simulink model "Robot_Sim"  (R2018a)
settings: Solver=ode45  StartTime=0.0  StopTime=Tsim  FixedStep=Ts_compute  RelTol=1e-3
values from neighbouring files (symbols this model uses):
  A_enc = [1 -Ts_sensor;0 1]    [Model.m]
  A_g = [1 -Ts_sensor;0 1]    [Model.m]
  A_y = [1 Ts_sensor Ts_sensor^2/2 ... (first row only)    [Model.m]
  B_enc = [Ts_sensor 0]'    [Model.m]
  B_g = [Ts_sensor 0]'    [Model.m]
  buffer_size = 15    [Model.m]
  C_enc = [1 0]    [Model.m]
  C_g = [1 0]    [Model.m]
  C_y = [0 0 1]    [Model.m]
  D_den = [1 2*D_WN*D_QSI D_WN^2]    [Model.m]
  D_num = D_WN^2    (= 81)    [Model.m]
  D_rodas = 0.4    [Model.m]
  Di_angle = pi/6    (= 0.523598775598)    [Model.m]
  Di_den = [1 2*Di_WN*Di_QSI Di_WN^2]    [Model.m]
  Di_num = Di_WN^2    (= 9)    [Model.m]
  Di_time = (2.5)*Tsim/8    (= 25)    [Model.m]
  discriminator = 0.8    [Model.m]
  g = u(7)    [ControllerK.m]    (also in Klankar_Marcus.m = 40; LQR.m = 40; Model.m = 40)
  Gyro_bias = 0.004    [Model.m]
  Kd = 0    [Model.m]
  Ki = 10.0    (= 10)    [Model.m]
  Kp = 5.0    (= 5)    [Model.m]
  ksi = u(6)    [ControllerK.m]    (also in Klankar_Marcus.m = 0.3; LQR.m = 0.3; Model.m = 0.6)
  Rv_enc = 0.002    [Model.m]
  Rv_g = 0.020    (= 0.02)    [Model.m]
  Rv_y = 0.01    [Model.m]
  Rw_enc = 0.1*[Ts_sensor^2/2 0;0 Ts_sensor^2/2]    [Model.m]
  Rw_g = 0.01*[Ts_sensor^2/2 0;0 Ts_sensor]    [Model.m]
  Rw_y = 0.05*[Ts_sensor^5/20 Ts_sensor^4/8 Ts_sensor^3/6 ... (first row only)    [Model.m]
  SELETOR_CONTROLADOR = 3    [Model.m]
  Time = 0:Ts:(time-1)*Ts    [InterfaceBT.m]
  Ts = 0.1    [InterfaceBT.m]    (also in Klankar_Marcus.m; LQR.m; Model.m)
  Ts_sensor = 1/50    (= 0.02)    [Model.m]
  Tsim = 70    [Klankar_Marcus.m]    (also in LQR.m = 63; Model.m = 80)
  V_MAX = 1    [Model.m]
  V_WHEEL_MAX = 1    [Model.m]
  W_MAX = 1    [Model.m]
undefined symbols (not defined in the file or in its folder): Controlador_LPV, DiscIntNeverNeededParam, Discrete, K_KALM_g, K_LQ
libraries: simulink x8, ctrlSharedLib x2, cstblocks x2
settings Model: PauseTimes=28  NumberOfSteps=10  Creator=davi2  LastModifiedBy=marcus
settings OptimizationCC: LifeSpan=inf
settings DebuggingCC: SFExecutionAtInitializationDiag=none
settings HardwareCC: ProdBitPerSizeT=32  ProdBitPerPtrDiffT=32  ProdWordSize=32  ProdHWDeviceType=Specified
settings CodeAppCC: StateflowObjectComments=on
settings SimscapeCC: SimscapeNormalizeSystem=off

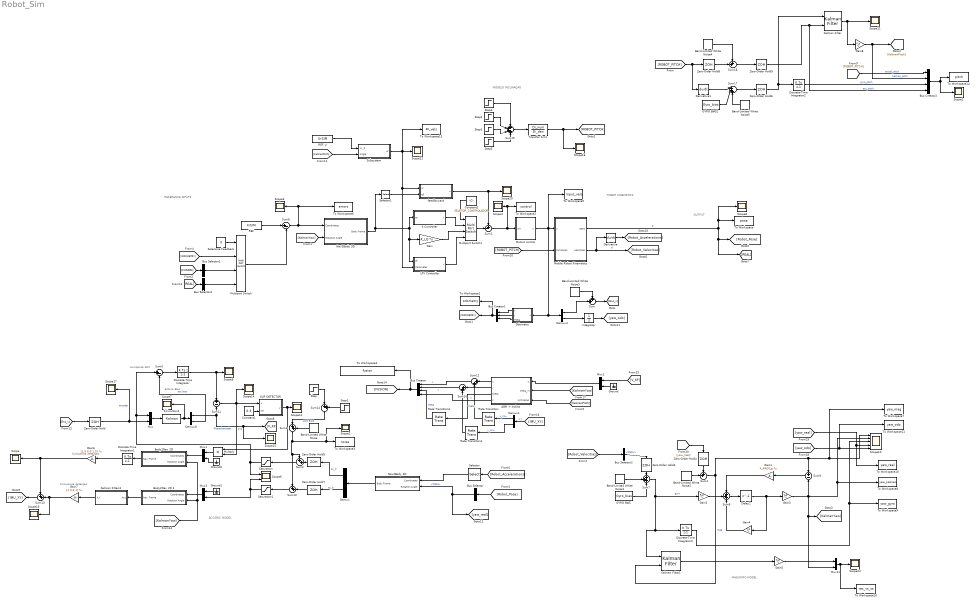
== system Robot_Sim ==
  note: MODELO INCLINAÇAO
  note: Compensa detecçao
  note: estima Bias
  note: compensa ACC
  note: OUTPUT
  note: ROBOT KINEMATICS
  note: MAG/GYRO MODEL
  note: ACC/ENC MODEL
  note: REFERENCE INPUTS
  note: Compensa detecçao
  AGM + Inclina : Subsystem
  Band-Limited White Noise : simulink/Sources/Band-Limited White Noise  Cov=Rv_y^2  Ts=Ts_sensor  seed=[23341]
  Band-Limited White Noise1 : simulink/Sources/Band-Limited White Noise  Cov=Rw_g(1,1)*Rw_g(1,1)  Ts=Ts_sensor  seed=[23341]
  Band-Limited White Noise2 : simulink/Sources/Band-Limited White Noise  Cov=Rv_g^2  Ts=Ts_sensor  seed=[23341]
  Band-Limited White Noise3 : simulink/Sources/Band-Limited White Noise  Cov=Rv_enc^2  Ts=Ts_sensor  seed=[23341]
  Band-Limited White Noise4 : simulink/Sources/Band-Limited White Noise  Cov=Rv_g^2  Ts=Ts_sensor  seed=[23341]
  Band-Limited White Noise5 : simulink/Sources/Band-Limited White Noise  Cov=Rw_g(1,1)*Rw_g(1,1)  Ts=Ts_sensor  seed=[23341]
  Body2Nav 2D : Subsystem
  Body2Nav 2D 2 : Subsystem
  Bus Creator : BusCreator  Inputs=4
  Bus Creator1 : BusCreator  Inputs=3
  Bus Creator2 : BusCreator  Inputs=4
  Bus Selector : BusSelector  OutputSignals=theta
  Bus Selector1 : BusSelector  OutputSignals=x,y,theta  OutputAsBus=on
  Bus Selector2 : BusSelector  OutputSignals=theta'
  Bus Selector3 : BusSelector  OutputSignals=x,y,theta  OutputAsBus=on
  Constant1 : Constant  Value=0.3
  Constant2 : Constant  Value=SELETOR_CONTROLADOR
  Delay2 : Delay  DelayLength=1
  Demux{,1,4,8} (4 alike) : Demux  Outputs=2
  Derivative : Derivative  CoefficientInTFapproximation=1
  Derivative1 : Derivative
  Discrete-Time Integrator : DiscreteIntegrator  IntegratorMethod=Integration: Backward Euler  SampleTime=Ts_sensor  ICPrevOutput=DiscIntNeverNeededParam  ICPrevScaledInput=DiscIntNeverNeededParam
  Discrete-Time Integrator1 : DiscreteIntegrator  SampleTime=Ts_sensor  ICPrevOutput=DiscIntNeverNeededParam  ICPrevScaledInput=DiscIntNeverNeededParam
  Discrete-Time Integrator2 : DiscreteIntegrator  SampleTime=-1  ICPrevOutput=DiscIntNeverNeededParam  ICPrevScaledInput=DiscIntNeverNeededParam
  Discrete-Time Integrator3 : DiscreteIntegrator  SampleTime=-1  ICPrevOutput=DiscIntNeverNeededParam  ICPrevScaledInput=DiscIntNeverNeededParam
  GYRO BIAS : Constant  Value=Gyro_bias
  GYRO BIAS1 : Constant  Value=Gyro_bias
  Gain : Gain  Gain=-K_LQ  Multiplication=Matrix(K*u)
  Gain1 : Gain  Gain=K_KALM_g  Multiplication=Matrix(K*u)
  Gain2 : Gain  Gain=B_g  Multiplication=Matrix(K*u)
  Gain3 : Gain  Gain=C_g  Multiplication=Matrix(K*u)
  Gain4 : Gain  Gain=A_g  Multiplication=Matrix(K*u)
  Gain5 : Gain  Gain=C_g  Multiplication=Matrix(K*u)
  Gain6 : Gain  Gain=[1.5 0;0 1.5]  Multiplication=Matrix(K*u)
  Gain7 : Gain  Gain=[1 0;0 1]  Multiplication=Matrix(K*u)
  Gain8 : Gain  Gain=C_g  Multiplication=Matrix(K*u)
  Ground : Ground
  Ground1 : Ground
  Ground2 : Ground
  Integrator : Integrator
  K Controller : Subsystem
  Kalman Filter : ctrlSharedLib/Kalman Filter  TimeDomain=Discrete-Time  UseCurrentEstimator=on  ModelSource=Individual A, B, C, D matrices  ModelSourceVariable=ss(0.95,1,1,0,1)  A=A_g  B=B_g  C=C_g  D=0  NumberOfStates=1  NumberOfInputs=1  NumberOfOutputs=1  InitialEstimateSource=Dialog  X0=0  P0=10  UseK=off  UseGH=off  NumberOfProcessNoiseInputs=1  G=1  TimeInvariantG=on  H=0  TimeInvariantH=on  Q=Rw_g  TimeInvariantQ=on  R=Rv_g  TimeInvariantR=on  N=0  TimeInvariantN=on  AddInputPort=on  AddEnablePort=off  OutputEstimatedY=off  OutputP=off  Ts=Ts_sensor
      settings: SourceProductBaseCode=CT
  Kalman Filter1 : ctrlSharedLib/Kalman Filter  TimeDomain=Discrete-Time  UseCurrentEstimator=on  ModelSource=LTI State-Space Variable  ModelSourceVariable=ss(A_g,B_g,C_g,0,Ts_sensor)  A=0.95  B=1  C=1  D=0  NumberOfStates=1  NumberOfInputs=1  NumberOfOutputs=1  InitialEstimateSource=Dialog  X0=0  P0=10  UseK=off  UseGH=off  NumberOfProcessNoiseInputs=1  G=1  TimeInvariantG=on  H=0  TimeInvariantH=on  Q=Rw_g  TimeInvariantQ=on  R=Rv_g  TimeInvariantR=on  N=0  TimeInvariantN=on  AddInputPort=on  AddEnablePort=off  OutputEstimatedY=off  OutputP=off  Ts=-1
      settings: SourceProductBaseCode=CT
  Kalman Filters1 : Subsystem
  "LPV Controller " : Subsystem
  Mobile Robot Kinematics : Subsystem
  Motors control : Subsystem
  Multiply : Product
  Multiport Switch : MultiPortSwitch
  Multiport Switch1 : MultiPortSwitch
  Mux{,1..3,11} (5 alike) : Mux  Inputs=2
  Nav2Body 2D : Subsystem
  Nav2Body 3D : Subsystem
  Odometry : Subsystem
  REF : FromWorkspace  VariableName=XrSIM  SampleTime=Ts  OutputAfterFinalValue=Holding final value
  REF U : FromWorkspace  VariableName=UrSIM  SampleTime=Ts  OutputAfterFinalValue=Holding final value
  Rate Transition : RateTransition  OutPortSampleTime=Ts
  Rate Transition1 : RateTransition  OutPortSampleTime=Ts
  Rate Transition3 : RateTransition  OutPortSampleTime=Ts
  S-Function2 : S-Function  FunctionName=Kalman  Parameters=Ts_sensor,A_enc,B_enc,C_enc,Rw_enc,Rv_enc  SFunctionDeploymentMode=off  EnableBusSupport=off
  SLIP DETECTOR : MATLAB Function  TreatAsAtomicUnit=on
  Saturation : Saturate  UpperLimit=4*9.8  LowerLimit=-4*9.8
  Saturation1 : Saturate  UpperLimit=4*9.8  LowerLimit=-4*9.8
  Scope{,1..5,7..8,11..12,14..17,19..21,24} (18 alike) : Scope
  Scope10 : Scope  NumInputPorts=5
  Scope6 : Scope  NumInputPorts=2
  Seleciona Feedback : Constant  Value=3
  Selector : Selector  InputPortWidth=3  IndexOptions=Index vector (dialog)  Indices=[1 2]  OutputSizes=1
  Selector1 : Selector  InputPortWidth=3  IndexOptions=Index vector (dialog)  Indices=3  OutputSizes=1
  Step : Step  Time=10  After=0.05  SampleTime=Ts_sensor
  Step1 : Step  Time=30  After=-0.05  SampleTime=Ts_sensor
  Step2 : Step  Time=Di_time+10  After=-Di_angle  SampleTime=0
  Step3 : Step  Time=Di_time+30  After=-Di_angle  SampleTime=0
  Step4 : Step  Time=Di_time  After=Di_angle  SampleTime=0
  Step5 : Step  Time=Di_time+42  After=Di_angle  SampleTime=0
  Subsystem : Subsystem
  Sum{,2,4,10,13,18} (6 alike) : Sum  Inputs=++|
  Sum1 : Sum  Inputs=+-|
  Sum11 : Sum  Inputs=+-
  Sum{3,12,14,16} (4 alike) : Sum  Inputs=|++
  Sum15 : Sum  Inputs=++++
  Sum17 : Sum  Inputs=|+++
  Sum5 : Sum  Inputs=|+-
  Sum6 : Sum  Inputs=|+-
  Sum7 : Sum  Inputs=+++
  Sum8 : Sum  Inputs=+++
  Sum9 : Sum  Inputs=+-
  To Workspace : ToWorkspace  VariableName=pose  SaveFormat=Timeseries  SampleTime=-1
  To Workspace1 : ToWorkspace  VariableName=odometry  SaveFormat=Timeseries  SampleTime=-1
  To Workspace10 : ToWorkspace  VariableName=yaw_real  SaveFormat=Timeseries  SampleTime=-1
  To Workspace11 : ToWorkspace  VariableName=yaw_odo  SaveFormat=Timeseries  SampleTime=-1
  To Workspace13 : ToWorkspace  VariableName=FF_vels  SaveFormat=Timeseries  SampleTime=-1
  To Workspace14 : ToWorkspace  VariableName=pitch  SaveFormat=Timeseries  SampleTime=-1
  To Workspace16 : ToWorkspace  VariableName=rec_vs_ss  SaveFormat=Timeseries  SampleTime=-1
  To Workspace2 : ToWorkspace  VariableName=control  SaveFormat=Timeseries  SampleTime=-1
  To Workspace3 : ToWorkspace  VariableName=noise  SaveFormat=Timeseries  SampleTime=-1
  To Workspace4 : ToWorkspace  VariableName=fusion  SaveFormat=Timeseries  SampleTime=-1
  To Workspace5 : ToWorkspace  VariableName=input_vels  SaveFormat=Timeseries  SampleTime=-1
  To Workspace6 : ToWorkspace  VariableName=errors  SaveFormat=Timeseries  SampleTime=-1
  To Workspace7 : ToWorkspace  VariableName=yaw_mag  SaveFormat=Timeseries  SampleTime=-1
  To Workspace8 : ToWorkspace  VariableName=yaw_kalman  SaveFormat=Timeseries  SampleTime=-1
  To Workspace9 : ToWorkspace  VariableName=yaw_gyro  SaveFormat=Timeseries  SampleTime=-1
  Transfer Fcn1 : TransferFcn  Numerator=Di_num  Denominator=Di_den
  Zero-Order Hold{,3..9} (8 alike) : ZeroOrderHold  SampleTime=Ts_sensor
  feedforward : Subsystem
  wires:
  Nav2Body 3D/1(Body Frame) -> "LPV Controller "/1(er), Gain/1, K Controller/1(er), Selector1/1
  Selector1/1 -> feedforward/2(e3)
  Motors control/1(u) -> Odometry/1(u), Demux4/1, Mobile Robot Kinematics/1(u), To Workspace5/1
  Sum1/1 -> Motors control/1(uin), To Workspace2/1, Scope4/1
  Band-Limited White Noise2/1 -> Sum4/2
  Demux/1 -> Zero-Order Hold5/1  "ax_b"
  Demux/2 -> Zero-Order Hold7/1  "ay_b"
  REF/1 -> Sum6/1
  Mobile Robot Kinematics/2(velocities) -> [Robot_Velocities], Derivative/1  "p'"
  Sum3/1 -> Scope2/1, To Workspace3/1, Sum2/1, Sum10/1
  Band-Limited White Noise/1 -> Sum3/2
  Sum14/1 -> Sum3/1  "ACC BIAS"
  Sum10/1 -> Saturation1/1
  Band-Limited White Noise1/1 -> Sum7/2
  GYRO BIAS/1 -> Sum7/3
  Sum7/1 -> Gain2/1, Kalman Filter1/1, Discrete-Time Integrator3/1  "gyro"
  Sum4/1 -> Kalman Filter1/2, Scope10/1, To Workspace7/1, Sum9/1  "mag"
  Sum8/1 -> Delay2/1
  Gain2/1 -> Sum8/2
  Delay2/1 -> Gain3/1, Gain4/1
  Gain4/1 -> Sum8/3
  Gain1/1 -> Sum8/1
  Gain3/1 -> Scope10/2, To Workspace8/1, Mux11/2, [KalmanYaw], Sum9/2
  Sum9/1 -> Gain1/1
  Discrete-Time Integrator3/1 -> Scope10/3, To Workspace9/1
  feedforward/1(u) -> Sum1/1, Scope20/1
  Gain/1 -> Multiport Switch1/3
  Nav2Body 2D/1(Body Frame) -> Demux/1
  [KalmanYaw] -> Nav2Body 3D/2(Rotation Angle)
  Sum6/1 -> Scope3/1, To Workspace6/1, Nav2Body 3D/1(Coordinates)
  Kalman Filter1/1 -> Gain5/1
  Mux11/1 -> To Workspace16/1, Scope24/1
  Gain5/1 -> Mux11/1
  [ODOMETRY] -> Multiport Switch/2
  Multiport Switch/1 -> Sum6/2
  Seleciona Feedback/1 -> Multiport Switch/1
  Demux4/2 -> Integrator/1
  [Robot_Pose] -> Bus Selector/1
  Mux3/1 -> Body2Nav 2D 2/1(Coordinates)
  Body2Nav 2D 2/1(Nav. Frame) -> Kalman Filters1/1(Acc)
  Bus Selector/1 -> [yaw_real], Nav2Body 2D/2(Rotation Angle)  "<theta>"
  [Robot_Velocities] -> Bus Selector2/1
  Zero-Order Hold3/1 -> Sum7/1
  Bus Selector2/1 -> Zero-Order Hold3/1  "<theta'>"
  Zero-Order Hold4/1 -> Sum4/1
  [KalmanYaw] -> Body2Nav 2D 2/2(Rotation Angle), Body2Nav 2D/2(Rotation Angle)
  [Enc_v] -> Zero-Order Hold/1
  Mux/1 -> S-Function2/1
  S-Function2/1 -> Scope7/1, Demux8/1
  Demux8/1 -> Scope15/1, [V_KF], Sum11/2  "filtered encoder"
  Demux8/2 -> Sum5/2  "acc bias"
  Discrete-Time Integrator/1 -> Sum11/1, Scope5/1
  Sum11/1 -> Scope14/1, Multiply/2, SLIP DETECTOR/1(u)  "slip"
  Constant1/1 -> SLIP DETECTOR/2(thr)
  Body2Nav 2D/1(Nav. Frame) -> Discrete-Time Integrator1/1
  Discrete-Time Integrator1/1 -> Gain6/1
  Zero-Order Hold/1 -> Scope17/1, Mux/2  "encoder"
  SLIP DETECTOR/1(y) -> Multiply/1, Scope12/1
  Mux1/1 -> Body2Nav 2D/1(Coordinates)
  Sum5/1 -> Discrete-Time Integrator/1
  Kalman Filters1/1(X,Y) -> Gain7/1
  Sum13/1 -> [IMU_XY]
  Ground1/1 -> Mux3/1
  Ground2/1 -> Mux1/2
  Multiply/1 -> Mux1/1
  Gain6/1 -> Sum13/1, Scope/1
  Gain7/1 -> Scope19/1, Sum13/2
  Step/1 -> Sum14/1
  Step1/1 -> Sum14/2
  Integrator/1 -> [yaw_odo]
  [yaw_odo] -> To Workspace11/1, Scope10/5
  [yaw_real] -> Zero-Order Hold4/1
  [yaw_real] -> To Workspace10/1, Scope10/4
  Saturation/1 -> Scope6/1, Mux/1, Sum5/1
  Saturation1/1 -> Mux3/2, Scope6/2
  Sum2/1 -> Saturation/1
  Zero-Order Hold7/1 -> Sum10/2
  Zero-Order Hold5/1 -> Sum2/2
  Derivative/1 -> [Robot_Accelerations]
  [Robot_Accelerations] -> Selector/1
  Selector/1 -> Nav2Body 2D/1(Coordinates)
  Mobile Robot Kinematics/1(pose) -> [Robot_Pose], [REAL], To Workspace/1, Scope8/1  "P"
  Transfer Fcn1/1 -> [ROBOT_PITCH], Scope16/1
  [KalmanYaw] -> AGM + Inclina/2(theta_in)
  Ground/1 -> Mux2/2
  [V_KF] -> Mux2/1
  Mux2/1 -> AGM + Inclina/1(u)
  Band-Limited White Noise3/1 -> Sum/1
  Demux4/1 -> Sum/2
  Sum/1 -> [Enc_v]
  Sum15/1 -> Transfer Fcn1/1
  Step4/1 -> Sum15/1
  [IMU_XY] -> Demux1/1  "x,y"
  AGM + Inclina/1(x) -> Sum12/1
  Demux1/1 -> Rate Transition/1  "x_imu"
  AGM + Inclina/2(y) -> Sum16/1
  Demux1/2 -> Rate Transition1/1  "y_imu"
  Sum12/1 -> Bus Creator/1  "x"
  Sum16/1 -> Bus Creator/2  "y"
  AGM + Inclina/4(z) -> Bus Creator/4  "z"
  Bus Creator/1 -> To Workspace4/1, [FUSION]
  [FUSION] -> Bus Selector1/1
  Bus Selector1/1 -> Multiport Switch/3
  Odometry/1(x) -> Bus Creator1/1
  Odometry/2(y) -> Bus Creator1/2
  Odometry/3(theta) -> Bus Creator1/3
  Bus Creator1/1 -> To Workspace1/1, [ODOMETRY]
  Rate Transition/1 -> Sum12/2
  Rate Transition1/1 -> Sum16/2
  Step2/1 -> Sum15/2
  Step3/1 -> Sum15/3
  Step5/1 -> Sum15/4
  REF U/1 -> Subsystem/1(Vr_0)
  Subsystem/1(ur) -> To Workspace13/1, Scope21/1, feedforward/1(ur), "LPV Controller "/2(Parameter)
  "LPV Controller "/1(v) -> Multiport Switch1/4
  K Controller/1(v) -> Multiport Switch1/2
  Constant2/1 -> Multiport Switch1/1
  Multiport Switch1/1 -> Sum1/2
  [KalmanPitch] -> Subsystem/2(Angle)
  [ROBOT_PITCH] -> Mobile Robot Kinematics/2(inclinaçao)
  [KalmanPitch] -> AGM + Inclina/3("Inclinacao ")
  AGM + Inclina/3(theta) -> Rate Transition3/1  "theta"
  Rate Transition3/1 -> Bus Creator/3  "theta"
  [REAL] -> Bus Selector3/1
  Bus Selector3/1 -> Multiport Switch/4
  [ROBOT_PITCH] -> Zero-Order Hold8/1, Derivative1/1
  Derivative1/1 -> Sum17/1
  GYRO BIAS1/1 -> Sum17/2
  Sum17/1 -> Zero-Order Hold6/1
  Zero-Order Hold6/1 -> Kalman Filter/1, Discrete-Time Integrator2/1
  Zero-Order Hold8/1 -> Sum18/2
  Band-Limited White Noise4/1 -> Sum18/1
  Sum18/1 -> Zero-Order Hold9/1
  Zero-Order Hold9/1 -> Bus Creator2/4, Kalman Filter/2  "acc_pitch"
  Kalman Filter/1 -> Gain8/1, Scope11/1
  Gain8/1 -> Bus Creator2/2, [KalmanPitch]  "kalman_pitch"
  [ROBOT_PITCH] -> Bus Creator2/1  "actual_pitch"
  Discrete-Time Integrator2/1 -> Bus Creator2/3  "gyro_pitch"
  Bus Creator2/1 -> Scope1/1, To Workspace14/1
  Band-Limited White Noise5/1 -> Sum17/3

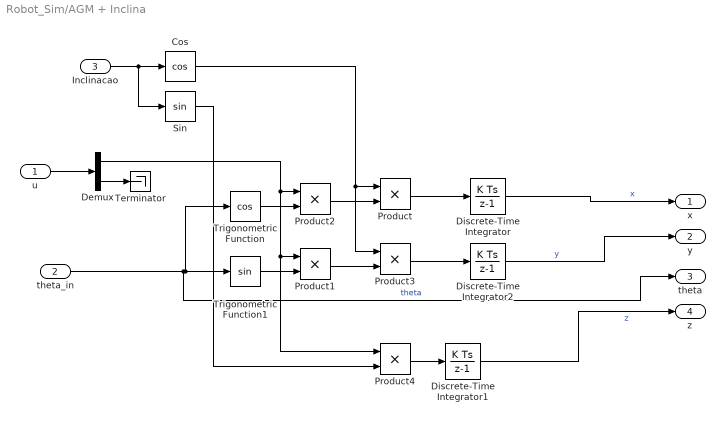
== system Robot_Sim/AGM + Inclina ==
  u : Inport
  theta_in : Inport  Port=2
  "Inclinacao " : Inport  Port=3
  Cos : Trigonometry  Operator=cos
  Demux : Demux  Outputs=2
  Discrete-Time Integrator : DiscreteIntegrator  SampleTime=Ts  ICPrevOutput=DiscIntNeverNeededParam  ICPrevScaledInput=DiscIntNeverNeededParam
  Discrete-Time Integrator1 : DiscreteIntegrator  SampleTime=Ts  ICPrevOutput=DiscIntNeverNeededParam  ICPrevScaledInput=DiscIntNeverNeededParam
  Discrete-Time Integrator2 : DiscreteIntegrator  SampleTime=Ts  ICPrevOutput=DiscIntNeverNeededParam  ICPrevScaledInput=DiscIntNeverNeededParam
  Product{,1..4} (5 alike) : Product
  Sin : Trigonometry
  Terminator : Terminator
  Trigonometric Function : Trigonometry  Operator=cos
  Trigonometric Function1 : Trigonometry
  x : Outport
  y : Outport  Port=2
  theta : Outport  Port=3
  z : Outport  Port=4
  wires:
  u/1 -> Demux/1
  Trigonometric Function/1 -> Product2/2
  Demux/1 -> Product4/1, Product1/1, Product2/1
  Trigonometric Function1/1 -> Product1/2
  Discrete-Time Integrator/1 -> x/1  "x"
  Discrete-Time Integrator2/1 -> y/1  "y"
  Demux/2 -> Terminator/1
  theta_in/1 -> theta/1, Trigonometric Function/1, Trigonometric Function1/1  "theta"
  "Inclinacao "/1 -> Sin/1, Cos/1
  Product2/1 -> Product/2
  Product1/1 -> Product3/2
  Cos/1 -> Product3/1, Product/1
  Product/1 -> Discrete-Time Integrator/1
  Product3/1 -> Discrete-Time Integrator2/1
  Sin/1 -> Product4/2
  Product4/1 -> Discrete-Time Integrator1/1
  Discrete-Time Integrator1/1 -> z/1  "z"

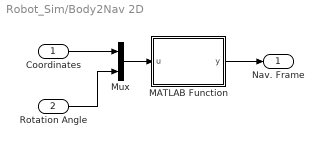
== system Robot_Sim/Body2Nav 2D ==
  Coordinates : Inport
  Rotation Angle : Inport  Port=2
  MATLAB Function : MATLAB Function  TreatAsAtomicUnit=on
  Mux : Mux  Inputs=2
  Nav. Frame : Outport
  wires:
  Coordinates/1 -> Mux/1
  Rotation Angle/1 -> Mux/2
  Mux/1 -> MATLAB Function/1(u)
  MATLAB Function/1(y) -> Nav. Frame/1

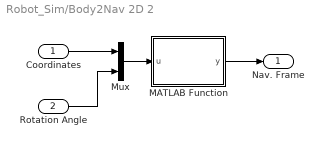
== system Robot_Sim/Body2Nav 2D 2 ==
  Coordinates : Inport
  Rotation Angle : Inport  Port=2
  MATLAB Function : MATLAB Function  TreatAsAtomicUnit=on
  Mux : Mux  Inputs=2
  Nav. Frame : Outport
  wires:
  Coordinates/1 -> Mux/1
  Rotation Angle/1 -> Mux/2
  Mux/1 -> MATLAB Function/1(u)
  MATLAB Function/1(y) -> Nav. Frame/1

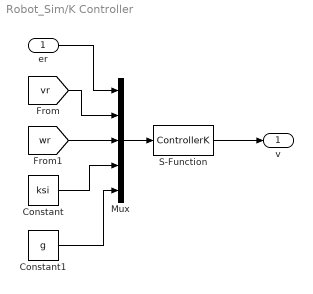
== system Robot_Sim/K Controller ==
  er : Inport
  Constant : Constant  Value=ksi
  Constant1 : Constant  Value=g
  Mux : Mux  Inputs=5
  S-Function : S-Function  FunctionName=ControllerK  Parameters=Ts  SFunctionDeploymentMode=off  EnableBusSupport=off
  v : Outport
  wires:
  er/1 -> Mux/1
  [vr] -> Mux/2
  [wr] -> Mux/3
  Constant/1 -> Mux/4
  Constant1/1 -> Mux/5
  Mux/1 -> S-Function/1
  S-Function/1 -> v/1

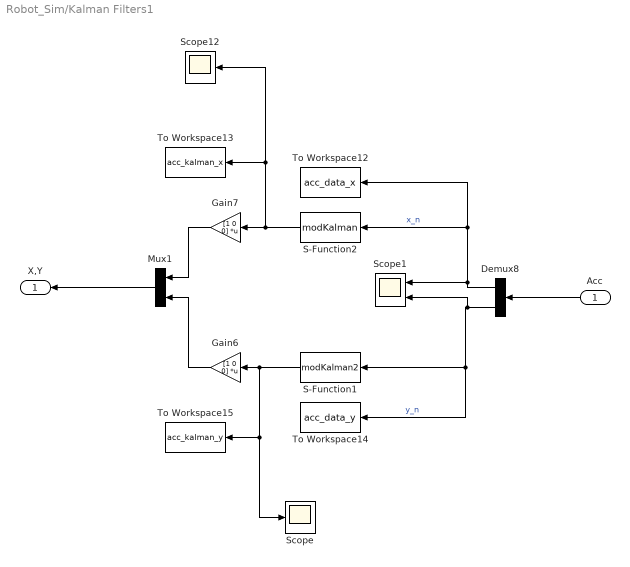
== system Robot_Sim/Kalman Filters1 ==
  Acc : Inport
  Demux8 : Demux  Outputs=2
  Gain6 : Gain  Gain=[1 0 0]  Multiplication=Matrix(K*u)
  Gain7 : Gain  Gain=[1 0 0]  Multiplication=Matrix(K*u)
  Mux1 : Mux  Inputs=2
  S-Function1 : S-Function  FunctionName=modKalman2  Parameters=Ts_sensor,A_y,C_y,Rw_y,Rv_y,discriminator,buffer_size  SFunctionDeploymentMode=off  EnableBusSupport=off
  S-Function2 : S-Function  FunctionName=modKalman  Parameters=Ts_sensor,A_y,C_y,Rw_y,Rv_y,discriminator,buffer_size  SFunctionDeploymentMode=off  EnableBusSupport=off
  Scope : Scope
  Scope1 : Scope  NumInputPorts=2
  Scope12 : Scope
  To Workspace12 : ToWorkspace  VariableName=acc_data_x  SaveFormat=Timeseries  SampleTime=-1
  To Workspace13 : ToWorkspace  VariableName=acc_kalman_x  SaveFormat=Timeseries  SampleTime=-1
  To Workspace14 : ToWorkspace  VariableName=acc_data_y  SaveFormat=Timeseries  SampleTime=-1
  To Workspace15 : ToWorkspace  VariableName=acc_kalman_y  SaveFormat=Timeseries  SampleTime=-1
  X,Y : Outport
  wires:
  Demux8/2 -> Scope1/2, S-Function1/1, To Workspace14/1  "y_n"
  S-Function2/1 -> To Workspace13/1, Scope12/1, Gain7/1
  Gain7/1 -> Mux1/1
  Demux8/1 -> Scope1/1, S-Function2/1, To Workspace12/1  "x_n"
  S-Function1/1 -> Scope/1, To Workspace15/1, Gain6/1
  Mux1/1 -> X,Y/1
  Gain6/1 -> Mux1/2
  Acc/1 -> Demux8/1

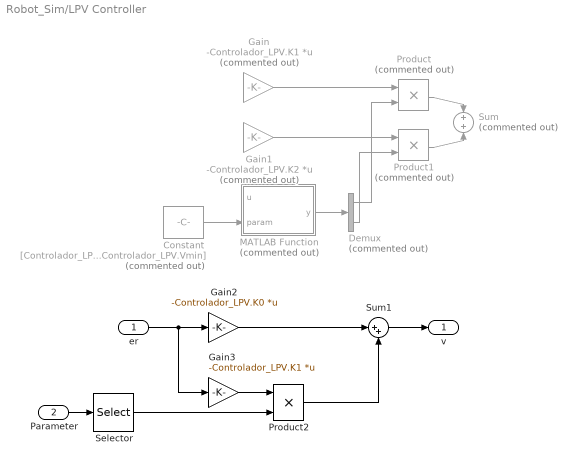
== system Robot_Sim/LPV Controller  ==
  er : Inport
  Parameter : Inport  Port=2
  Constant : Constant  Commented=on  Value=[Controlador_LPV.Vmax Controlador_LPV.Vmin]
  Demux : Demux  Commented=on  Outputs=2
  Gain : Gain  Commented=on  Gain=-Controlador_LPV.K1  Multiplication=Matrix(K*u)
  Gain1 : Gain  Commented=on  Gain=-Controlador_LPV.K2  Multiplication=Matrix(K*u)
  Gain2 : Gain  Gain=-Controlador_LPV.K0  Multiplication=Matrix(K*u)
  Gain3 : Gain  Gain=-Controlador_LPV.K1  Multiplication=Matrix(K*u)
  MATLAB Function : MATLAB Function  Commented=on  TreatAsAtomicUnit=on
  Product : Product  Commented=on
  Product1 : Product  Commented=on
  Product2 : Product
  Selector : Selector  InputPortWidth=2  IndexOptions=Index vector (dialog)  Indices=1  OutputSizes=1
  Sum : Sum  Commented=on
  Sum1 : Sum  Inputs=|++
  v : Outport
  wires:
  Gain/1 -> Product/1
  Gain1/1 -> Product1/1
  Demux/1 -> Product/2
  Demux/2 -> Product1/2
  Product/1 -> Sum/1
  Product1/1 -> Sum/2
  MATLAB Function/1(y) -> Demux/1
  Constant/1 -> MATLAB Function/2(param)
  Gain3/1 -> Product2/1
  er/1 -> Gain2/1, Gain3/1
  Gain2/1 -> Sum1/1
  Sum1/1 -> v/1
  Parameter/1 -> Selector/1
  Selector/1 -> Product2/2
  Product2/1 -> Sum1/2

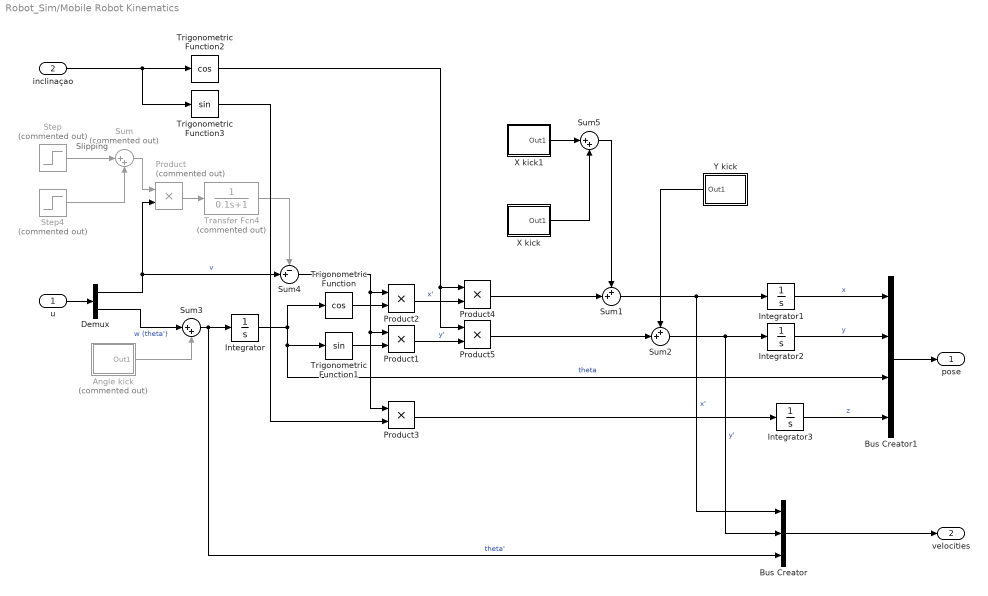
== system Robot_Sim/Mobile Robot Kinematics ==
  note: Slipping
  u : Inport
  inclinaçao : Inport  Port=2
  Angle kick : Subsystem  Commented=on  mask{T=3*Tsim/8, A=0.5}
      mask prompts: T "Time"; A "Amplitude"
      mask DialogControl DescTextVar Prompt: Applies a kick with 'Amplitude' at 'Time'
      mask Display: disp('Kick')
  Bus Creator : BusCreator  Inputs=3
  Bus Creator1 : BusCreator  Inputs=4
  Demux : Demux  Outputs=2
  Integrator{,1..3} (4 alike) : Integrator
  Product : Product  Commented=on
  Product{1..5} (5 alike) : Product
  Step : Step  Commented=on  Time=25  SampleTime=0
  Step4 : Step  Commented=on  Time=27  After=-1  SampleTime=0
  Sum : Sum  Commented=on  Inputs=|++
  Sum1 : Sum  Inputs=++|
  Sum2 : Sum  Inputs=++|
  Sum3 : Sum  Inputs=|++
  Sum4 : Sum  Inputs=-+|
  Sum5 : Sum  Inputs=|++
  Transfer Fcn4 : TransferFcn  Commented=on  Numerator=1  Denominator=[0.1 1]
  Trigonometric Function : Trigonometry  Operator=cos
  Trigonometric Function1 : Trigonometry
  Trigonometric Function2 : Trigonometry  Operator=cos
  Trigonometric Function3 : Trigonometry
  X kick : Subsystem  mask{T=70, A=1}
      mask prompts: T "Time"; A "Amplitude"
      mask DialogControl DescTextVar Prompt: Applies a kick with 'Amplitude' at 'Time'
      mask Display: disp('Kick')
  X kick1 : Subsystem  mask{T=30, A=1}
      mask prompts: T "Time"; A "Amplitude"
      mask DialogControl DescTextVar Prompt: Applies a kick with 'Amplitude' at 'Time'
      mask Display: disp('Kick')
  Y kick : Subsystem  mask{T=50, A=1}
      mask prompts: T "Time"; A "Amplitude"
      mask DialogControl DescTextVar Prompt: Applies a kick with 'Amplitude' at 'Time'
      mask Display: disp('Kick')
  pose : Outport
  velocities : Outport  Port=2
  wires:
  u/1 -> Demux/1
  Trigonometric Function/1 -> Product2/2
  Demux/1 -> Sum4/2, Product/2  "v"
  Trigonometric Function1/1 -> Product1/2
  Bus Creator1/1 -> pose/1
  Integrator/1 -> Bus Creator1/3, Trigonometric Function1/1, Trigonometric Function/1  "theta"
  Step/1 -> Sum/1
  Step4/1 -> Sum/2
  Sum/1 -> Product/1
  Sum4/1 -> Product3/1, Product1/1, Product2/1
  Product/1 -> Transfer Fcn4/1
  Transfer Fcn4/1 -> Sum4/1
  Bus Creator/1 -> velocities/1
  Integrator2/1 -> Bus Creator1/2  "y"
  Integrator1/1 -> Bus Creator1/1  "x"
  Sum2/1 -> Bus Creator/2, Integrator2/1  "y'"
  Sum3/1 -> Bus Creator/3, Integrator/1  "theta'"
  Demux/2 -> Sum3/1  "w (theta')"
  Angle kick/1(Out1) -> Sum3/2
  Sum1/1 -> Bus Creator/1, Integrator1/1  "x'"
  Y kick/1(Out1) -> Sum2/1
  inclinaçao/1 -> Trigonometric Function3/1, Trigonometric Function2/1
  Integrator3/1 -> Bus Creator1/4  "z"
  Product3/1 -> Integrator3/1
  Trigonometric Function3/1 -> Product3/2
  Product2/1 -> Product4/2  "x'"
  Product1/1 -> Product5/2  "y'"
  Trigonometric Function2/1 -> Product5/1, Product4/1
  Product4/1 -> Sum1/2
  Product5/1 -> Sum2/2
  X kick1/1(Out1) -> Sum5/1
  X kick/1(Out1) -> Sum5/2
  Sum5/1 -> Sum1/1

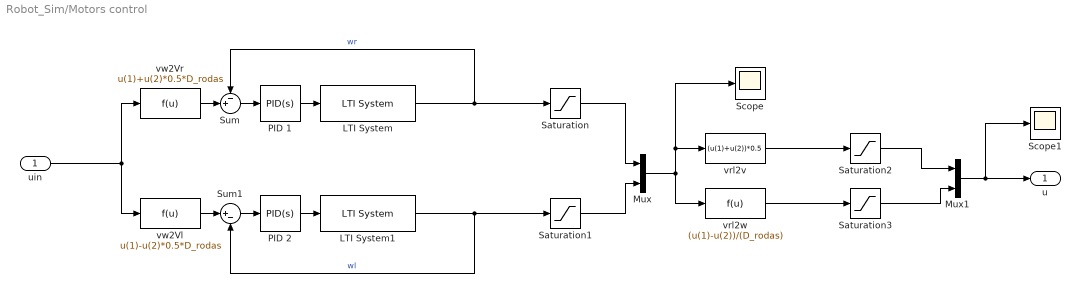
== system Robot_Sim/Motors control ==
  uin : Inport
  LTI System : cstblocks/LTI System  sys=HMotor  IC=[]
  LTI System1 : cstblocks/LTI System  sys=HMotor  IC=[]
  Mux : Mux  Inputs=2
  Mux1 : Mux  Inputs=2
  PID 1 : simulink/Continuous/PID Controller  Controller=PID  TimeDomain=Continuous-time  SampleTime=-1  IntegratorMethod=Forward Euler  FilterMethod=Forward Euler  Form=Parallel  UseFilter=on  ControllerParametersSource=internal  P=Kp  I=Ki  D=Kd  N=100  InitialConditionSource=internal  InitialConditionForIntegrator=0  InitialConditionForFilter=0  ExternalReset=none  LimitOutput=off  UpperSaturationLimit=inf  LowerSaturationLimit=-inf  LinearizeAsGain=on  AntiWindupMode=none  Kb=1  TrackingMode=off  Kt=1  PParamMin=[]  PParamMax=[]  IParamMin=[]  IParamMax=[]  DParamMin=[]  DParamMax=[]  NParamMin=[]  NParamMax=[]  KbParamMin=[]  KbParamMax=[]  KtParamMin=[]  KtParamMax=[]  POutMin=[]  POutMax=[]  IOutMin=[]  IOutMax=[]  DOutMin=[]  DOutMax=[]  NOutMin=[]  NOutMax=[]  KbOutMin=[]  KbOutMax=[]  KtOutMin=[]  KtOutMax=[]  IntegratorOutMin=[]  IntegratorOutMax=[]  FilterOutMin=[]  FilterOutMax=[]  SumOutMin=[]  SumOutMax=[]  SumI1OutMin=[]  SumI1OutMax=[]  SumI2OutMin=[]  SumI2OutMax=[]  SumI3OutMin=[]  SumI3OutMax=[]  SumDOutMin=[]  SumDOutMax=[]  SaturationOutMin=[]  SaturationOutMax=[]  IntegratorContinuousStateAttributes=''  IntegratorStateMustResolveToSignalObject=off  IntegratorRTWStateStorageClass=Auto  FilterContinuousStateAttributes=''  FilterStateMustResolveToSignalObject=off  FilterRTWStateStorageClass=Auto  DifferentiatorICPrevScaledInput=0  DifferentiatorOutMin=[]  DifferentiatorOutMax=[]  FilterDiffOutCoefMin=[]  FilterDiffOutCoefMax=[]  SumDenOutMin=[]  SumDenOutMax=[]  SumNumOutMin=[]  SumNumOutMax=[]  ReciprocalOutMin=[]  ReciprocalOutMax=[]  DivideOutMin=[]  DivideOutMax=[]  TunerSelectOption=Transfer Function Based (PID Tuner App)
  PID 2 : simulink/Continuous/PID Controller  Controller=PID  TimeDomain=Continuous-time  SampleTime=-1  IntegratorMethod=Forward Euler  FilterMethod=Forward Euler  Form=Parallel  UseFilter=on  ControllerParametersSource=internal  P=Kp  I=Ki  D=Kd  N=100  InitialConditionSource=internal  InitialConditionForIntegrator=0  InitialConditionForFilter=0  ExternalReset=none  LimitOutput=off  UpperSaturationLimit=inf  LowerSaturationLimit=-inf  LinearizeAsGain=on  AntiWindupMode=none  Kb=1  TrackingMode=off  Kt=1  PParamMin=[]  PParamMax=[]  IParamMin=[]  IParamMax=[]  DParamMin=[]  DParamMax=[]  NParamMin=[]  NParamMax=[]  KbParamMin=[]  KbParamMax=[]  KtParamMin=[]  KtParamMax=[]  POutMin=[]  POutMax=[]  IOutMin=[]  IOutMax=[]  DOutMin=[]  DOutMax=[]  NOutMin=[]  NOutMax=[]  KbOutMin=[]  KbOutMax=[]  KtOutMin=[]  KtOutMax=[]  IntegratorOutMin=[]  IntegratorOutMax=[]  FilterOutMin=[]  FilterOutMax=[]  SumOutMin=[]  SumOutMax=[]  SumI1OutMin=[]  SumI1OutMax=[]  SumI2OutMin=[]  SumI2OutMax=[]  SumI3OutMin=[]  SumI3OutMax=[]  SumDOutMin=[]  SumDOutMax=[]  SaturationOutMin=[]  SaturationOutMax=[]  IntegratorContinuousStateAttributes=''  IntegratorStateMustResolveToSignalObject=off  IntegratorRTWStateStorageClass=Auto  FilterContinuousStateAttributes=''  FilterStateMustResolveToSignalObject=off  FilterRTWStateStorageClass=Auto  DifferentiatorICPrevScaledInput=0  DifferentiatorOutMin=[]  DifferentiatorOutMax=[]  FilterDiffOutCoefMin=[]  FilterDiffOutCoefMax=[]  SumDenOutMin=[]  SumDenOutMax=[]  SumNumOutMin=[]  SumNumOutMax=[]  ReciprocalOutMin=[]  ReciprocalOutMax=[]  DivideOutMin=[]  DivideOutMax=[]  TunerSelectOption=Transfer Function Based (PID Tuner App)
  Saturation : Saturate  UpperLimit=V_WHEEL_MAX  LowerLimit=-V_WHEEL_MAX
  Saturation1 : Saturate  UpperLimit=V_WHEEL_MAX  LowerLimit=-V_WHEEL_MAX
  Saturation2 : Saturate  UpperLimit=V_MAX  LowerLimit=0
  Saturation3 : Saturate  UpperLimit=W_MAX  LowerLimit=-W_MAX
  Scope : Scope
  Scope1 : Scope
  Sum : Sum  Inputs=-+|
  Sum1 : Sum  Inputs=|+-
  vrl2v : Fcn  Expr=(u(1)+u(2))*0.5
  vrl2w : Fcn  Expr=(u(1)-u(2))/(D_rodas)
  vw2Vl : Fcn  Expr=u(1)-u(2)*0.5*D_rodas
  vw2Vr : Fcn  Expr=u(1)+u(2)*0.5*D_rodas
  u : Outport
  wires:
  LTI System1/1 -> Saturation1/1, Sum1/2  "wl"
  vw2Vl/1 -> Sum1/1
  Sum1/1 -> PID 2/1
  PID 2/1 -> LTI System1/1
  Sum/1 -> PID 1/1
  PID 1/1 -> LTI System/1
  LTI System/1 -> Saturation/1, Sum/1  "wr"
  uin/1 -> vw2Vr/1, vw2Vl/1
  Mux/1 -> vrl2w/1, Scope/1, vrl2v/1
  Mux1/1 -> Scope1/1, u/1
  vrl2v/1 -> Saturation2/1
  vrl2w/1 -> Saturation3/1
  vw2Vr/1 -> Sum/2
  Saturation/1 -> Mux/1
  Saturation1/1 -> Mux/2
  Saturation2/1 -> Mux1/1
  Saturation3/1 -> Mux1/2

== system Robot_Sim/Nav2Body 2D ==
  Coordinates : Inport
  Rotation Angle : Inport  Port=2
  MATLAB Function : MATLAB Function  TreatAsAtomicUnit=on
  Mux : Mux  Inputs=2
  Body Frame : Outport
  wires:
  Coordinates/1 -> Mux/1
  Rotation Angle/1 -> Mux/2
  Mux/1 -> MATLAB Function/1(u)
  MATLAB Function/1(y) -> Body Frame/1

== system Robot_Sim/Nav2Body 3D ==
  Coordinates : Inport
  Rotation Angle : Inport  Port=2
  MATLAB Function : MATLAB Function  TreatAsAtomicUnit=on
  Mux : Mux  Inputs=2
  Body Frame : Outport
  wires:
  Coordinates/1 -> Mux/1
  Rotation Angle/1 -> Mux/2
  Mux/1 -> MATLAB Function/1(u)
  MATLAB Function/1(y) -> Body Frame/1

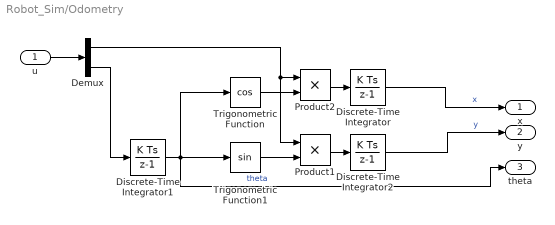
== system Robot_Sim/Odometry ==
  u : Inport
  Demux : Demux  Outputs=2
  Discrete-Time Integrator : DiscreteIntegrator  SampleTime=Ts  ICPrevOutput=DiscIntNeverNeededParam  ICPrevScaledInput=DiscIntNeverNeededParam
  Discrete-Time Integrator1 : DiscreteIntegrator  SampleTime=Ts  ICPrevOutput=DiscIntNeverNeededParam  ICPrevScaledInput=DiscIntNeverNeededParam
  Discrete-Time Integrator2 : DiscreteIntegrator  SampleTime=Ts  ICPrevOutput=DiscIntNeverNeededParam  ICPrevScaledInput=DiscIntNeverNeededParam
  Product1 : Product
  Product2 : Product
  Trigonometric Function : Trigonometry  Operator=cos
  Trigonometric Function1 : Trigonometry
  x : Outport
  y : Outport  Port=2
  theta : Outport  Port=3
  wires:
  u/1 -> Demux/1
  Demux/2 -> Discrete-Time Integrator1/1
  Trigonometric Function/1 -> Product2/2
  Demux/1 -> Product1/1, Product2/1
  Product2/1 -> Discrete-Time Integrator/1
  Trigonometric Function1/1 -> Product1/2
  Product1/1 -> Discrete-Time Integrator2/1
  Discrete-Time Integrator/1 -> x/1  "x"
  Discrete-Time Integrator2/1 -> y/1  "y"
  Discrete-Time Integrator1/1 -> theta/1, Trigonometric Function1/1, Trigonometric Function/1  "theta"

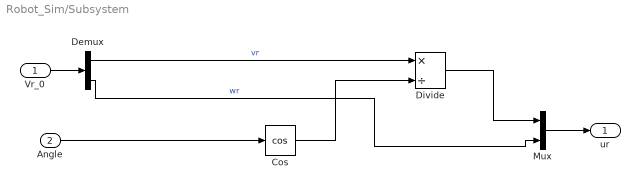
== system Robot_Sim/Subsystem ==
  Vr_0 : Inport
  Angle : Inport  Port=2
  Cos : Trigonometry  Operator=cos
  Demux : Demux  Outputs=2
  Divide : Product  Inputs=*/
  Mux : Mux  Inputs=2
  ur : Outport
  wires:
  Vr_0/1 -> Demux/1
  Mux/1 -> ur/1
  Angle/1 -> Cos/1
  Demux/2 -> Mux/2  "wr"
  Divide/1 -> Mux/1
  Demux/1 -> Divide/1  "vr"
  Cos/1 -> Divide/2

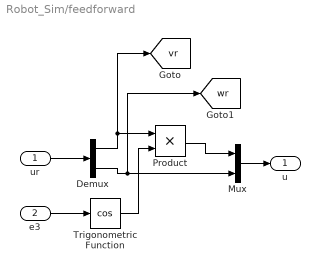
== system Robot_Sim/feedforward ==
  ur : Inport
  e3 : Inport  Port=2
  Demux : Demux  Outputs=2
  Mux : Mux  Inputs=2
  Product : Product
  Trigonometric Function : Trigonometry  Operator=cos
  u : Outport
  tag scope: vr=global, wr=global
  wires:
  e3/1 -> Trigonometric Function/1
  ur/1 -> Demux/1
  Demux/1 -> [vr], Product/1
  Trigonometric Function/1 -> Product/2
  Product/1 -> Mux/1
  Demux/2 -> [wr], Mux/2
  Mux/1 -> u/1

== system Robot_Sim/Mobile Robot Kinematics/Angle kick ==
  Step : Step  Time=T  After=2*A  SampleTime=0
  Step1 : Step  Time=T+0.5  After=-2*A  SampleTime=0
  Sum : Sum
  Transfer Fcn1 : TransferFcn  Numerator=D_num  Denominator=D_den
  Out1 : Outport
  wires:
  Step/1 -> Sum/1
  Step1/1 -> Sum/2
  Sum/1 -> Transfer Fcn1/1
  Transfer Fcn1/1 -> Out1/1

== system Robot_Sim/Mobile Robot Kinematics/X kick ==
  Step : Step  Time=T  After=2*A  SampleTime=0
  Step1 : Step  Time=T+0.5  After=-2*A  SampleTime=0
  Sum : Sum
  Transfer Fcn1 : TransferFcn  Numerator=D_num  Denominator=D_den
  Out1 : Outport
  wires:
  Step/1 -> Sum/1
  Step1/1 -> Sum/2
  Sum/1 -> Transfer Fcn1/1
  Transfer Fcn1/1 -> Out1/1

== system Robot_Sim/Mobile Robot Kinematics/X kick1 ==
  Step : Step  Time=T  After=2*A  SampleTime=0
  Step1 : Step  Time=T+0.5  After=-2*A  SampleTime=0
  Sum : Sum
  Transfer Fcn1 : TransferFcn  Numerator=D_num  Denominator=D_den
  Out1 : Outport
  wires:
  Step/1 -> Sum/1
  Step1/1 -> Sum/2
  Sum/1 -> Transfer Fcn1/1
  Transfer Fcn1/1 -> Out1/1

== system Robot_Sim/Mobile Robot Kinematics/Y kick ==
  Step : Step  Time=T  After=2*A  SampleTime=0
  Step1 : Step  Time=T+0.5  After=-2*A  SampleTime=0
  Sum : Sum
  Transfer Fcn1 : TransferFcn  Numerator=D_num  Denominator=D_den
  Out1 : Outport
  wires:
  Step/1 -> Sum/1
  Step1/1 -> Sum/2
  Sum/1 -> Transfer Fcn1/1
  Transfer Fcn1/1 -> Out1/1

== matlab function Robot_Sim/Nav2Body 3D/MATLAB Function ==
  data: u input; y output
function y = fcn(u)

roation = u(4);

M = [cos(roation) sin(roation) 0;
     -sin(roation) cos(roation) 0;
     0 0 1];
 
y = M*[u(1) u(2) u(3)]';

== matlab function Robot_Sim/Nav2Body 2D/MATLAB Function ==
  data: u input; y output
function y = fcn(u)
rotation = u(3);

M = [cos(rotation) sin(rotation);
     -sin(rotation) cos(rotation)];
 
y = M*[u(1) u(2)]';

== matlab function Robot_Sim/SLIP DETECTOR ==
  data: u input; y output; thr input
function y = fcn(u,thr)
if(u > thr || u<-thr)
    y = 1;
else
    y = 0;
end

== matlab function Robot_Sim/Body2Nav 2D/MATLAB Function ==
  data: u input; y output
function y = fcn(u)
rotation = u(3);

M = [cos(rotation) -sin(rotation);
     sin(rotation) cos(rotation)];
 
y = M*[u(1) u(2)]';

== matlab function Robot_Sim/LPV Controller /MATLAB Function ==
  data: u input; y output; param input
function y = fcn(u,param)
coder.extrinsic('evalin');
vr = u(1);
% ab = evalin('base','Controlador_LPV.Vmax');
vr_max = param(1);
vr_min = param(2);
den = (vr_max - vr_min);
beta1 = (vr_max - vr)/den;
beta2 = (vr - vr_min)/den;
y = [beta1 beta2]';

== matlab function Robot_Sim/Body2Nav 2D 2/MATLAB Function ==
  data: u input; y output
function y = fcn(u)
rotation = u(3);

M = [cos(rotation) -sin(rotation);
     sin(rotation) cos(rotation)];
 
y = M*[u(1) u(2)]';
